simulink model "Lab3_varios_alfas"  (R2020b)
settings: Solver=VariableStepAuto  StartTime=0.0  StopTime=20  MaxStep=1e-2  RelTol=1e-3
libraries: simulink x5
settings Model: Creator=rodsc  LastModifiedBy=rodsc
settings SolverCC: ZeroCrossAlgorithm=Adaptive
settings DebuggingCC: IgnoredZcDiagnostic=none

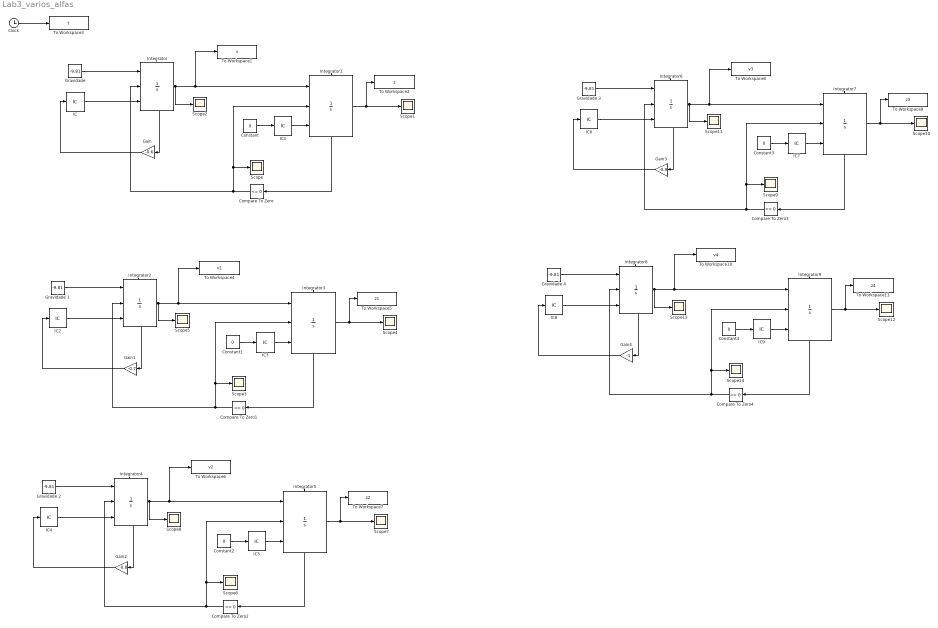
== system Lab3_varios_alfas ==
  Clock : Clock
  Compare To Zero{,1..4} (5 alike) : simulink/Logic and Bit Operations/Compare To Zero  relop=<=  OutDataTypeStr=boolean
  Constant{,1..4} (5 alike) : Constant  Value=0
  Gain : Gain  Gain=-0.6
  Gain1 : Gain  Gain=-0.7
  Gain2 : Gain  Gain=-0.8
  Gain3 : Gain  Gain=-0.9
  Gain4 : Gain  Gain=-1
  Gravidade {,1..4} (5 alike) : Constant  Value=-9.81
  IC{,2,4,6,8} (5 alike) : InitialCondition  Value=0
  IC{1,3,5,7,9} (5 alike) : InitialCondition  Value=10
  Integrator{,2,4,6,8} (5 alike) : Integrator  ExternalReset=rising  InitialConditionSource=external  ShowStatePort=on
  Integrator{1,3,5,7,9} (5 alike) : Integrator  ExternalReset=rising  InitialConditionSource=external  LowerSaturationLimit=0  ShowStatePort=on
  Scope{,1..14} (15 alike) : Scope
  To Workspace1 : ToWorkspace  VariableName=v  SampleTime=-1
      settings: Save2DSignal=2-D array (concatenate along first dimension)
  To Workspace10 : ToWorkspace  VariableName=v4  SampleTime=-1
      settings: Save2DSignal=2-D array (concatenate along first dimension)
  To Workspace11 : ToWorkspace  VariableName=z4  SampleTime=-1
      settings: Save2DSignal=2-D array (concatenate along first dimension)
  To Workspace2 : ToWorkspace  VariableName=z  SampleTime=-1
      settings: Save2DSignal=2-D array (concatenate along first dimension)
  To Workspace3 : ToWorkspace  VariableName=t  SampleTime=-1
      settings: Save2DSignal=2-D array (concatenate along first dimension)
  To Workspace4 : ToWorkspace  VariableName=v1  SampleTime=-1
      settings: Save2DSignal=2-D array (concatenate along first dimension)
  To Workspace5 : ToWorkspace  VariableName=z1  SampleTime=-1
      settings: Save2DSignal=2-D array (concatenate along first dimension)
  To Workspace6 : ToWorkspace  VariableName=v2  SampleTime=-1
      settings: Save2DSignal=2-D array (concatenate along first dimension)
  To Workspace7 : ToWorkspace  VariableName=z2  SampleTime=-1
      settings: Save2DSignal=2-D array (concatenate along first dimension)
  To Workspace8 : ToWorkspace  VariableName=v3  SampleTime=-1
      settings: Save2DSignal=2-D array (concatenate along first dimension)
  To Workspace9 : ToWorkspace  VariableName=z3  SampleTime=-1
      settings: Save2DSignal=2-D array (concatenate along first dimension)
  wires:
  "Gravidade "/1 -> Integrator/1
  IC/1 -> Integrator/3
  Integrator/1 -> Scope2/1, To Workspace1/1, Integrator1/1
  Gain/1 -> IC/1
  Integrator/State -> Gain/1
  Integrator1/State -> Compare To Zero/1
  Compare To Zero/1 -> Integrator/2, Scope/1, Integrator1/2
  Constant/1 -> IC1/1
  IC1/1 -> Integrator1/3
  Integrator1/1 -> To Workspace2/1, Scope1/1
  Clock/1 -> To Workspace3/1
  IC3/1 -> Integrator3/3
  Integrator3/1 -> To Workspace5/1, Scope4/1
  IC2/1 -> Integrator2/3
  Integrator3/State -> Compare To Zero1/1
  Integrator2/State -> Gain1/1
  Constant1/1 -> IC3/1
  Gain1/1 -> IC2/1
  Integrator2/1 -> Scope5/1, To Workspace4/1, Integrator3/1
  Compare To Zero1/1 -> Integrator2/2, Scope3/1, Integrator3/2
  Gravidade 1/1 -> Integrator2/1
  IC5/1 -> Integrator5/3
  Integrator5/1 -> To Workspace7/1, Scope7/1
  IC4/1 -> Integrator4/3
  Integrator5/State -> Compare To Zero2/1
  Integrator4/State -> Gain2/1
  Constant2/1 -> IC5/1
  Gain2/1 -> IC4/1
  Integrator4/1 -> Scope8/1, To Workspace6/1, Integrator5/1
  Compare To Zero2/1 -> Integrator4/2, Scope6/1, Integrator5/2
  Gravidade 2/1 -> Integrator4/1
  IC7/1 -> Integrator7/3
  Integrator7/1 -> To Workspace9/1, Scope10/1
  IC6/1 -> Integrator6/3
  Integrator7/State -> Compare To Zero3/1
  Integrator6/State -> Gain3/1
  Constant3/1 -> IC7/1
  Gain3/1 -> IC6/1
  Integrator6/1 -> Scope11/1, To Workspace8/1, Integrator7/1
  Compare To Zero3/1 -> Integrator6/2, Scope9/1, Integrator7/2
  Gravidade 3/1 -> Integrator6/1
  Gravidade 4/1 -> Integrator8/1
  Compare To Zero4/1 -> Integrator8/2, Scope14/1, Integrator9/2
  Integrator8/1 -> Scope13/1, To Workspace10/1, Integrator9/1
  Constant4/1 -> IC9/1
  Integrator8/State -> Gain4/1
  Gain4/1 -> IC8/1
  Integrator9/State -> Compare To Zero4/1
  IC8/1 -> Integrator8/3
  IC9/1 -> Integrator9/3
  Integrator9/1 -> To Workspace11/1, Scope12/1
